simulink model "SMC_Arduino"  (R2024b)
settings: Solver=FixedStepDiscrete  StartTime=0.0  StopTime=Inf  FixedStep=Ts_SMC_Arduino  RelTol=1e-3  EnableMultiTasking=on
undefined symbols (not defined in the file or in its folder): a_smc_equiv, alpha_mrac, beta_eq_smc, control_enable_SMC, gamma_mrac, gm_smc, gyro_bias_dps_SMC, gyro_sign_SMC, Ts_MRAC_Arduino, u_max_MRAC, u_min_MRAC
libraries: arduinolib x2, arduinosensorlib x1
settings Model: ExtModeTrigDuration=2  Creator=juanm  LastModifiedBy=juanm
settings SolverCC: AutoInsertRateTranBlk=on
settings OptimizationCC: EnhancedBackFolding=on  PassReuseOutputArgsAs=Individual arguments  ZeroExternalMemoryAtStartup=off  ZeroInternalMemoryAtStartup=off  MaxStackSize=64  OptimizeBlockOrder=speed  DifferentSizesBufferReuse=on  OptimizationCustomize=off  EfficientTunableParamExpr=on
settings DebuggingCC: ParameterTunabilityLossMsg=error
settings HardwareCC: ProdBitPerInt=16  ProdBitPerPointer=16  ProdBitPerSizeT=16  ProdBitPerPtrDiffT=16  ProdLargestAtomicFloat=None  ProdWordSize=8  ProdHWDeviceType=Atmel->AVR  UseEmbeddedCoderFeatures=off  UseSimulinkCoderFeatures=off
settings SFSimCC: MATLABDynamicMemAlloc=off
settings RTWCC: Description=Embedded Coder  SystemTargetFile=ert.tlc  HardwareBoard=Arduino Uno  TemplateMakefile=ert_default_tmf  Toolchain=Arduino AVR  BuildConfiguration=Faster Runs
settings CodeAppCC: ForceParamTrailComments=on  IgnoreCustomStorageClasses=off  OperatorAnnotations=on  SimulinkDataObjDesc=on  SFDataObjDesc=on  InsertBlockDesc=on
settings ERTTargetCC: SupportContinuousTime=on  SupportNonInlinedSFcns=on  SupportVariableSizeSignals=on  ExtModeTransport=3  ExtModeStaticAlloc=on  ExtModeAutomaticAllocSize=off  ExtModeStaticAllocSize=250  ExtModeMexFile=ext_xcp  ExtModeIntrfLevel=Level2 - Open  InlinedParameterPlacement=Hierarchical

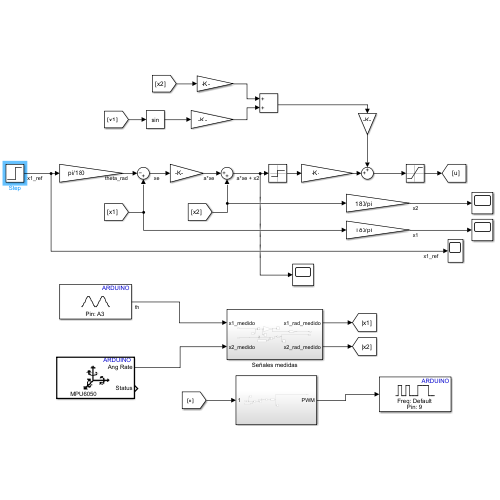
[thumbnail: Simulink's stored preview of the top-level diagram]
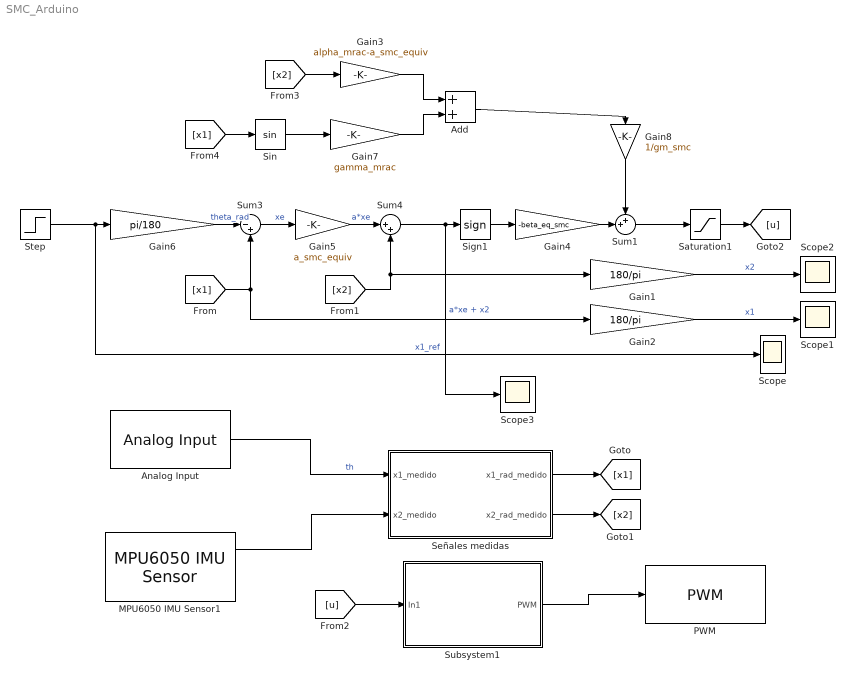
== system SMC_Arduino ==
  Add : Sum
  Analog Input : arduinolib/Analog Input  pinNumber=3  ReadResultsOnly=off  ConversionTriggerSource=Software  ExternalTriggerType=uint32( 0 )  OutputDataType=uint16  EnableConversionCompleteNotify=off  EnableOuputStatus=off  SampleTime=-1  blockPlatform=arduino
      settings: SourceProductName=Common
  Gain1 : Gain  Gain=180/pi
  Gain2 : Gain  Gain=180/pi
  Gain3 : Gain  Gain=alpha_mrac-a_smc_equiv
  Gain4 : Gain  Gain=-beta_eq_smc
  Gain5 : Gain  Gain=a_smc_equiv
  Gain6 : Gain  Gain=pi/180
  Gain7 : Gain  Gain=gamma_mrac
  Gain8 : Gain  Gain=1/gm_smc
  MPU6050 IMU Sensor1 : arduinosensorlib/MPU6050 IMU Sensor  I2CModule=0  SlaveAddress=0x68  Accel=off  AngularRate=on  Temperature=off  Status=on  Timestamp=off  EulerAngles=off  Quat=off  AccelRange=2G  GyroRange=250 dps  DmpOdr=200 Hz  Dlpf=Accelerometer: 184Hz, Gyroscope: 188Hz  spf=1  SampleTime=Ts_MRAC_Arduino  QueueSizeFactor=1
      settings: SourceProductName=Sensors
  PWM : arduinolib/PWM  pinNumber=9  frequencyType=Default  desiredFrequency=490.2  achievableFrequency=490.2
      settings: SourceProductName=Common
  Saturation1 : Saturate  UpperLimit=100  LowerLimit=0  ZeroCross=off
  Scope{,1..3} (4 alike) : Scope
  Señales medidas : Subsystem
  Sign1 : Signum  ZeroCross=off
  Sin : Trigonometry
  Step : Step  After=150  SampleTime=0
  Subsystem1 : Subsystem
  Sum1 : Sum  Inputs=++|
  Sum3 : Sum  Inputs=|-+
  Sum4 : Sum  Inputs=|++
  wires:
  Analog Input/1 -> Señales medidas/1(x1_medido)  "th"
  MPU6050 IMU Sensor1/1 -> Señales medidas/2(x2_medido)
  Subsystem1/1(PWM) -> PWM/1
  Sign1/1 -> Gain4/1
  Sum3/1 -> Gain5/1  "xe"
  Gain5/1 -> Sum4/1  "a*xe"
  Sum4/1 -> Scope3/1, Sign1/1  "a*xe + x2"
  Gain4/1 -> Sum1/2
  Step/1 -> Scope/1, Gain6/1  "x1_ref"
  Señales medidas/2(x2_rad_medido) -> [x2]
  Señales medidas/1(x1_rad_medido) -> [x1]
  [x1] -> Gain2/1, Sum3/2
  [x2] -> Gain1/1, Sum4/2
  Saturation1/1 -> [u]
  [u] -> Subsystem1/1(In1)
  Gain6/1 -> Sum3/1  "theta_rad"
  Gain2/1 -> Scope1/1  "x1"
  Gain1/1 -> Scope2/1  "x2"
  Gain3/1 -> Add/1
  [x1] -> Sin/1
  Sin/1 -> Gain7/1
  Add/1 -> Gain8/1
  Gain7/1 -> Add/2
  [x2] -> Gain3/1
  Sum1/1 -> Saturation1/1
  Gain8/1 -> Sum1/1

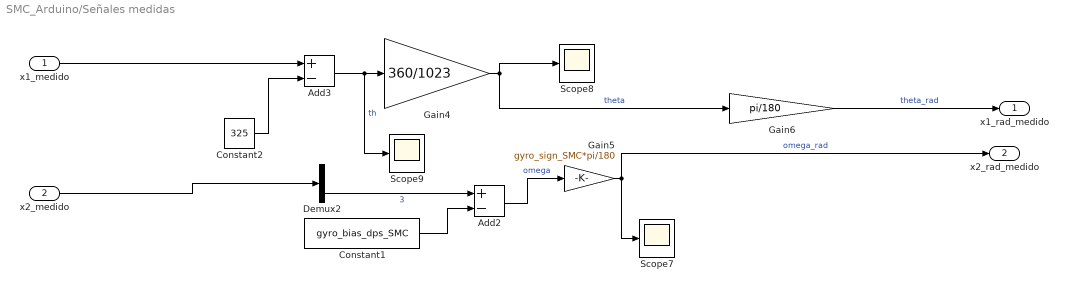
== system SMC_Arduino/Señales medidas ==
  x1_medido : Inport
  x2_medido : Inport  Port=2
  Add2 : Sum  Inputs=+-
  Add3 : Sum  Inputs=+-
  Constant1 : Constant  Value=gyro_bias_dps_SMC
  Constant2 : Constant  Value=325
  Demux2 : Demux  Outputs=3
  Gain4 : Gain  Gain=360/1023
  Gain5 : Gain  Gain=gyro_sign_SMC*pi/180
  Gain6 : Gain  Gain=pi/180
  Scope7 : Scope
  Scope8 : Scope
  Scope9 : Scope
  x1_rad_medido : Outport
  x2_rad_medido : Outport  Port=2
  wires:
  Add3/1 -> Scope9/1, Gain4/1  "th"
  Gain6/1 -> x1_rad_medido/1  "theta_rad"
  Gain4/1 -> Gain6/1, Scope8/1  "theta"
  Demux2/3 -> Add2/1  "3"
  x1_medido/1 -> Add3/1
  Gain5/1 -> x2_rad_medido/1, Scope7/1  "omega_rad"
  Constant1/1 -> Add2/2
  x2_medido/1 -> Demux2/1
  Add2/1 -> Gain5/1  "omega"
  Constant2/1 -> Add3/2

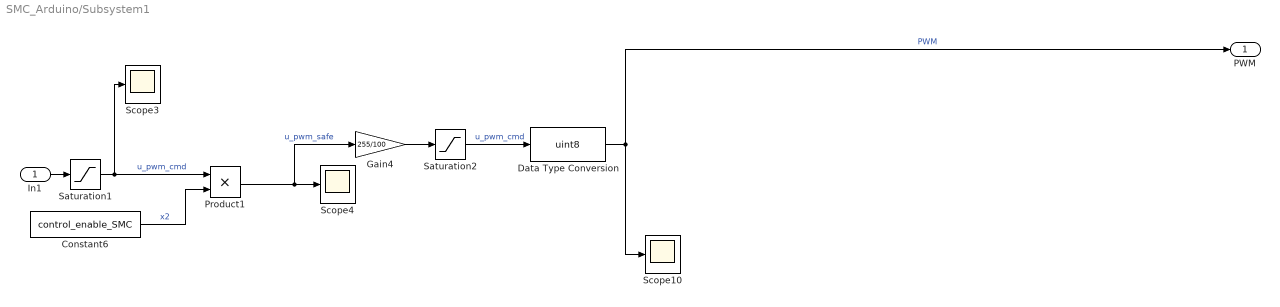
== system SMC_Arduino/Subsystem1 ==
  In1 : Inport
  Constant6 : Constant  Value=control_enable_SMC  VectorParams1D=off
  Data Type Conversion : DataTypeConversion  OutDataTypeStr=uint8  SaturateOnIntegerOverflow=off  RndMeth=Floor
  Gain4 : Gain  Gain=255/100
  Product1 : Product
  Saturation1 : Saturate  UpperLimit=u_max_MRAC  LowerLimit=u_min_MRAC
  Saturation2 : Saturate  UpperLimit=255  LowerLimit=0
  Scope10 : Scope
  Scope3 : Scope
  Scope4 : Scope
  PWM : Outport
  wires:
  Gain4/1 -> Saturation2/1
  Saturation1/1 -> Scope3/1, Product1/1  "u_pwm_cmd"
  Constant6/1 -> Product1/2  "x2"
  In1/1 -> Saturation1/1
  Saturation2/1 -> Data Type Conversion/1  "u_pwm_cmd"
  Product1/1 -> Gain4/1, Scope4/1  "u_pwm_safe"
  Data Type Conversion/1 -> PWM/1, Scope10/1  "PWM"
